simulink model "Demo_LQR_HSD_second"  (R2017a)
settings: Solver=ode1  StartTime=0.0  StopTime=30  FixedStep=0.001  RelTol=1e-3
undefined symbols (not defined in the file): K
settings Model: Creator=Lenovo  LastModifiedBy=307
settings DataIOCC: LimitDataPoints=on  SaveFormat=Array
settings OptimizationCC: BlockReduction=off  BooleanDataType=off  LifeSpan=inf
settings DebuggingCC: SaveWithParameterizedLinksMsg=none  UnderspecifiedInitializationDetection=Classic  MergeDetectMultiDrivingBlocksExec=none  SignalResolutionControl=TryResolveAllWithWarning  SFUnexpectedBacktrackingDiag=warning  SFNoUnconditionalDefaultTransitionDiag=warning  SFExecutionAtInitializationDiag=none
settings HardwareCC: ProdBitPerPointer=32  ProdBitPerSizeT=32  ProdBitPerPtrDiffT=32  ProdLargestAtomicFloat=None  ProdIntDivRoundTo=Undefined  ProdEndianess=Unspecified  ProdWordSize=32  ProdHWDeviceType=32-bit Generic  TargetUnknown=on
settings ModelReferenceCC: PropagateSignalLabelsOutOfModel=off
settings GRTTargetCC: TargetLangStandard=C89/C90 (ANSI)  GeneratePreprocessorConditionals=Disable all
settings ConfigComp: CovMetricSettings=dw  CovHtmlReporting=on  CovSaveCumulativeToWorkspaceVar=on  CovSaveSingleToWorkspaceVar=on  CovExternalEMLEnable=off  CovSFcnEnable=off

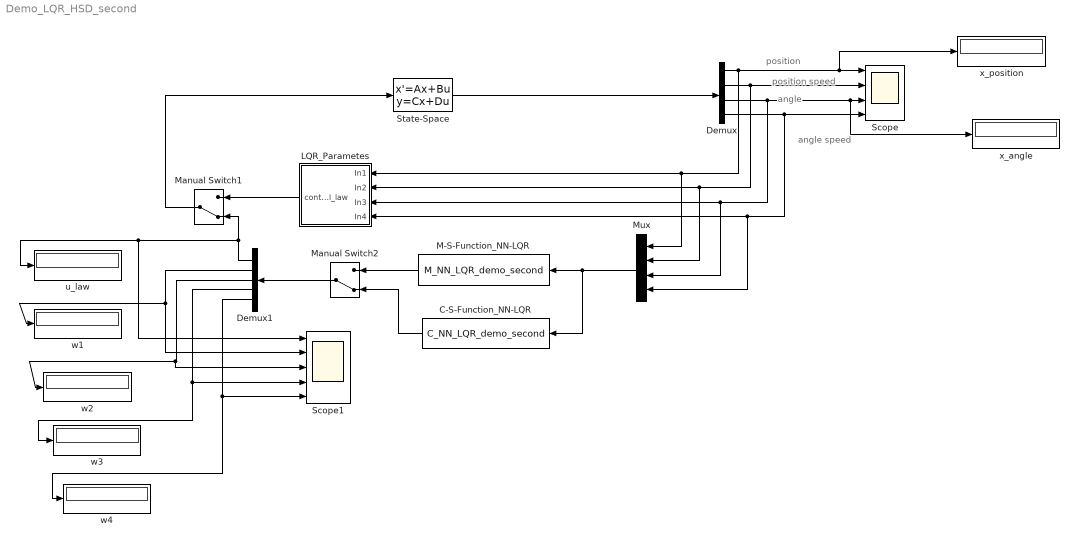
== system Demo_LQR_HSD_second ==
  note: angle speed
  note: angle
  note: position speed
  note: position
  C-S-Function_NN-LQR : S-Function  FunctionName=C_NN_LQR_demo_second  SFunctionDeploymentMode=off  EnableBusSupport=off
  Demux : Demux
  Demux1 : Demux  Outputs=5
  LQR_Parametes : Subsystem
  M-S-Function_NN-LQR : S-Function  FunctionName=M_NN_LQR_demo_second  SFunctionDeploymentMode=off  EnableBusSupport=off
  Manual Switch1 : ManualSwitch  CurrentSetting=0
  Manual Switch2 : ManualSwitch  CurrentSetting=0
  Mux : Mux
  Scope : Scope  NumInputPorts=4
  Scope1 : Scope  NumInputPorts=5
  State-Space : StateSpace  A=[0 1 0 0;0 -0.1164 1.2373 0;0 0 0 1;0 -0.7164 67.9221 0]  B=[0;1.4554;0;8.9546]  C=[1 0 0 0;0 1 0 0;0 0 1 0;0 0 0 1]  D=[0;0;0;0]  X0=[1;1;1;1]
  u_law : Display
  w{1..4} (4 alike) : Display
  x_angle : Display
  x_position : Display
  wires:
  State-Space/1 -> Demux/1
  Demux/1 -> LQR_Parametes/1(In1), Mux/1, x_position/1, Scope/1
  Demux/2 -> LQR_Parametes/2(In2), Mux/2, Scope/2
  Demux/4 -> LQR_Parametes/4(In4), Mux/4, Scope/4
  LQR_Parametes/1(control_law) -> Manual Switch1/1
  Demux/3 -> LQR_Parametes/3(In3), Mux/3, x_angle/1, Scope/3
  Demux1/1 -> Manual Switch1/2, Scope1/1, u_law/1
  Manual Switch1/1 -> State-Space/1
  Demux1/2 -> Scope1/2, w1/1
  Demux1/3 -> Scope1/3, w2/1
  Demux1/4 -> Scope1/4, w3/1
  Demux1/5 -> w4/1, Scope1/5
  Manual Switch2/1 -> Demux1/1
  M-S-Function_NN-LQR/1 -> Manual Switch2/1
  C-S-Function_NN-LQR/1 -> Manual Switch2/2
  Mux/1 -> C-S-Function_NN-LQR/1, M-S-Function_NN-LQR/1

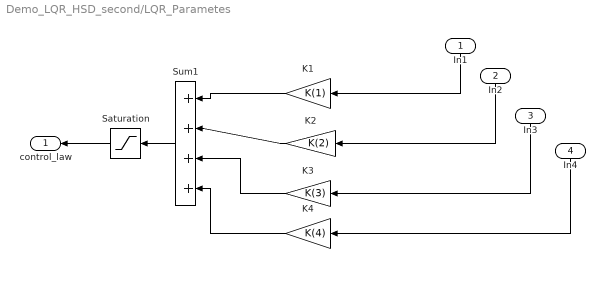
== system Demo_LQR_HSD_second/LQR_Parametes ==
  In1 : Inport
  In2 : Inport  Port=2
  In3 : Inport  Port=3
  In4 : Inport  Port=4
  K1 : Gain  Gain=K(1)
  K2 : Gain  Gain=K(2)
  K3 : Gain  Gain=K(3)
  K4 : Gain  Gain=K(4)
  Saturation : Saturate  UpperLimit=10  LowerLimit=-10
  Sum1 : Sum  Inputs=|++++
  control_law : Outport
  wires:
  In1/1 -> K1/1
  In3/1 -> K3/1
  In4/1 -> K4/1
  In2/1 -> K2/1
  K2/1 -> Sum1/2
  K1/1 -> Sum1/1
  K3/1 -> Sum1/3
  K4/1 -> Sum1/4
  Sum1/1 -> Saturation/1
  Saturation/1 -> control_law/1
